simulink model "MPC_mobile_base_KIN"  (R2018b)
settings: Solver=ode4  StartTime=0.0  StopTime=inf  FixedStep=Tsample  RelTol=1e-3
values from neighbouring files (symbols this model uses):
  N = 6    [MPC_kin_N=6arc traj.mat]    (also in MPC_kin_N=7complex traj_ultimo.mat = 7; MPC_kin_Param_N=10 traj_retta.mat = 10; MPC_kin_Param_N=10 traj_ultimo.mat = 10; Traj_Prova.m = 5)
  p_0 = [0 0 0 0 0 0 0]    [MPC_kin_Param_N=10 traj_retta.mat]    (also in MPC_kin_Param_N=10 traj_ultimo.mat; Traj_Prova.m = zeros(1,7); traiettoria2.m = zeros(1,7); untitled5.m = zeros(1,7))
  T = 0.5    [MPC_kin_N=6arc traj.mat]    (also in MPC_kin_N=7complex traj_ultimo.mat = 0.2; MPC_kin_Param_N=10 traj_retta.mat = 0.4; MPC_kin_Param_N=10 traj_ultimo.mat = 0.4; Traj_Prova.m = 0.2)
  Tsample = 0.01    [MPC_kin_N=6arc traj.mat]    (also in MPC_kin_N=7complex traj_ultimo.mat; MPC_kin_Param_N=10 traj_retta.mat; MPC_kin_Param_N=10 traj_ultimo.mat = 0.08; Traj_Prova.m)
  xd = [0 0 0 0 0 0.000654498469498 0.0758636207458 4.96526307585e-05 0.00261799387799 0.227590374774 0.000446873251435 0.00589048622548 ... (153 elements, 3x51)]    [MPC_kin_N=6arc traj.mat]    (also in MPC_kin_N=7complex traj_ultimo.mat = [0 0 0 0.1 0 0 0.2 0 0 0.3 0 0 ... (303 elements, 3x101)]; MPC_kin_Param_N=10 traj_retta.mat = [0 2 0.785398163397 0.08 2.08 0.785398163397 0.16 2.16 0.785; MPC_kin_Param_N=10 traj_ultimo.mat = [0 2 0.785398163397 0.016 2.016 0.785398163397 0.032 2.032 0; Traj_Prova.m = [xdx; xdy; xdth])
undefined symbols (not defined in the file or in its folder): DiscIntNeverNeededParam
libraries: simulink x3, templibrary x1
settings Model: Creator=RaffaelePC  LastModifiedBy=Francesco Gennari
settings DebuggingCC: UnderSpecifiedDimensionMsg=warning

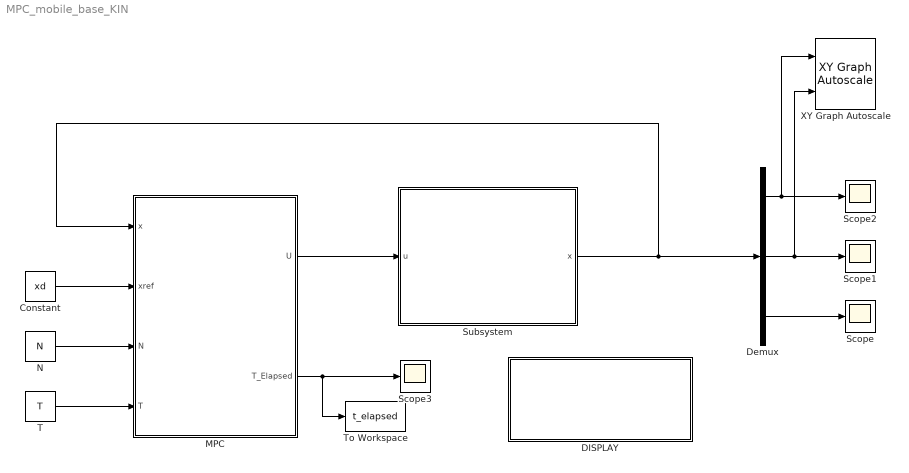
== system MPC_mobile_base_KIN ==
  Constant : Constant  Value=xd
  DISPLAY : Subsystem
  Demux : Demux  Outputs=3
  MPC : Subsystem
      mask Display: fprintf('MPC CONTROLLER')
  N : Constant  Value=N
  Scope{,1..3} (4 alike) : Scope
  Subsystem : Subsystem
      mask Display: disp('{\bf\fontsize{10}KINEMATIC SYSTEM}', 'texmode','on');
  T : Constant  Value=T
  To Workspace : ToWorkspace  VariableName=t_elapsed  SampleTime=T
      settings: Save2DSignal=2-D array (concatenate along first dimension)
  XY Graph Autoscale : templibrary/XY Graph  Autoscale  xmin=-1  xmax=1  ymin=-1  ymax=1  st=-1
  wires:
  N/1 -> MPC/3(N)
  T/1 -> MPC/4(T)
  Constant/1 -> MPC/2(xref)
  Subsystem/1(x) -> Demux/1, MPC/1(x)
  Demux/3 -> Scope/1
  Demux/1 -> XY Graph Autoscale/1, Scope2/1
  Demux/2 -> XY Graph Autoscale/2, Scope1/1
  MPC/2(T_Elapsed) -> To Workspace/1, Scope3/1
  MPC/1(U) -> Subsystem/1(u)

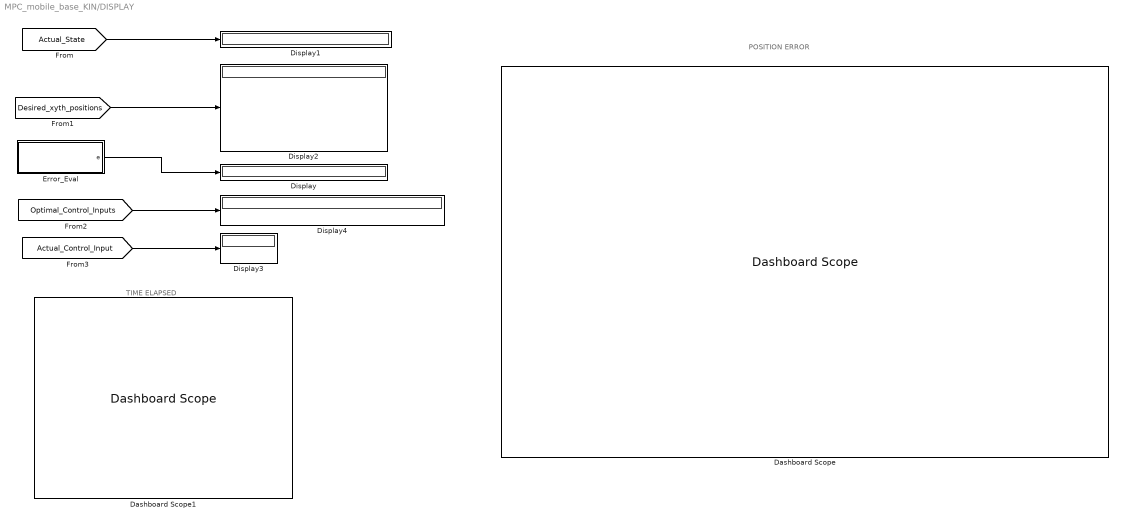
== system MPC_mobile_base_KIN/DISPLAY ==
  note: POSITION ERROR
  note: TIME ELAPSED
  Dashboard Scope : DashboardScope  WebBlockId=507  Ymin=-0.5  Ymax=0.5
  Dashboard Scope1 : DashboardScope  WebBlockId=516  Ymin=0  Ymax=1
  Display{,1..4} (5 alike) : Display
  "Error_Eval " : Subsystem
  wires:
  [Optimal_Control_Inputs] -> Display4/1
  [Desired_xyth_positions] -> Display2/1
  [Actual_Control_Input] -> Display3/1
  [Actual_State] -> Display1/1
  "Error_Eval "/1(e) -> Display/1

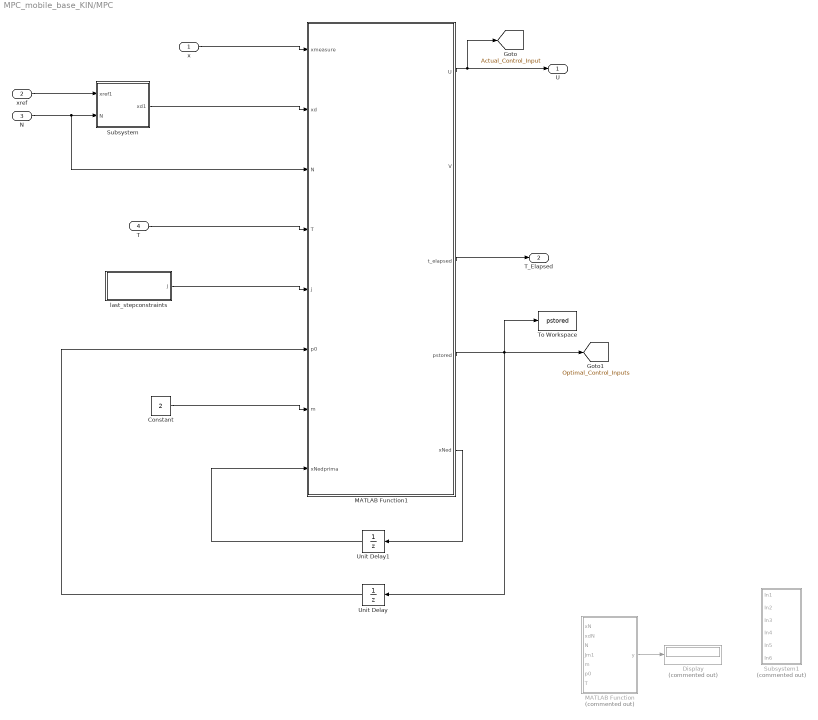
== system MPC_mobile_base_KIN/MPC ==
  x : Inport
  xref : Inport  Port=2
  N : Inport  Port=3
  T : Inport  Port=4
  Constant : Constant  Value=2
  Display : Display  Commented=on
  MATLAB Function : MATLAB Function  Commented=on  TreatAsAtomicUnit=on
  MATLAB Function1 : MATLAB Function  TreatAsAtomicUnit=on
  Subsystem : Subsystem
  Subsystem1 : Subsystem  Commented=on
  To Workspace : ToWorkspace  VariableName=pstored  SampleTime=-1
      settings: Save2DSignal=2-D array (concatenate along first dimension)
  Unit Delay : UnitDelay  InitialCondition=[0 0 0 0 0 0 N]  SampleTime=-1
  Unit Delay1 : UnitDelay  InitialCondition=zeros(2,3)  SampleTime=-1
  last_stepconstraints : Subsystem
  U : Outport
  T_Elapsed : Outport  Port=2
  tag scope: Actual_Control_Input=global, Optimal_Control_Inputs=global
  wires:
  Subsystem/1(xd1) -> MATLAB Function1/2(xd)
  MATLAB Function1/1(U) -> [Actual_Control_Input], U/1
  MATLAB Function1/4(pstored) -> [Optimal_Control_Inputs], To Workspace/1, Unit Delay/1
  Unit Delay/1 -> MATLAB Function1/6(p0)
  xref/1 -> Subsystem/1(xref1)
  x/1 -> MATLAB Function1/1(xmeasure)
  N/1 -> MATLAB Function1/3(N), Subsystem/2(N)
  T/1 -> MATLAB Function1/4(T)
  last_stepconstraints/1(j) -> MATLAB Function1/5(j)
  MATLAB Function1/3(t_elapsed) -> T_Elapsed/1
  MATLAB Function/1(y) -> Display/1
  Constant/1 -> MATLAB Function1/7(m)
  MATLAB Function1/5(xNed) -> Unit Delay1/1
  Unit Delay1/1 -> MATLAB Function1/8(xNedprima)

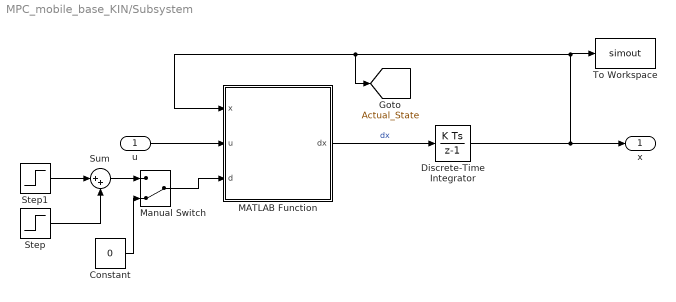
== system MPC_mobile_base_KIN/Subsystem ==
  u : Inport
  Constant : Constant  Value=0
  Discrete-Time Integrator : DiscreteIntegrator  InitialCondition=[0 0 0]  SampleTime=-1  ICPrevOutput=DiscIntNeverNeededParam  ICPrevScaledInput=DiscIntNeverNeededParam
  MATLAB Function : MATLAB Function  TreatAsAtomicUnit=on
  Manual Switch : ManualSwitch  CurrentSetting=0
  Step : Step  Time=100  SampleTime=Tsample
  Step1 : Step  Time=104  After=-1  SampleTime=Tsample
  Sum : Sum  Inputs=|++
  To Workspace : ToWorkspace  VariableName=simout  SaveFormat=Timeseries  SampleTime=-1
  x : Outport
  tag scope: Actual_State=global
  wires:
  u/1 -> MATLAB Function/2(u)
  MATLAB Function/1(dx) -> Discrete-Time Integrator/1  "dx"
  Discrete-Time Integrator/1 -> [Actual_State], MATLAB Function/1(x), To Workspace/1, x/1
  Step1/1 -> Sum/1
  Step/1 -> Sum/2
  Sum/1 -> Manual Switch/1
  Manual Switch/1 -> MATLAB Function/3(d)
  Constant/1 -> Manual Switch/2

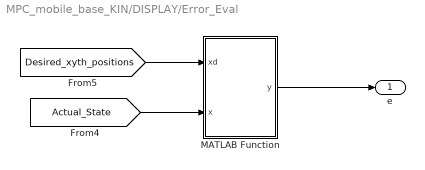
== system MPC_mobile_base_KIN/DISPLAY/Error_Eval  ==
  MATLAB Function : MATLAB Function  TreatAsAtomicUnit=on
  e : Outport
  wires:
  MATLAB Function/1(y) -> e/1
  [Desired_xyth_positions] -> MATLAB Function/1(xd)
  [Actual_State] -> MATLAB Function/2(x)

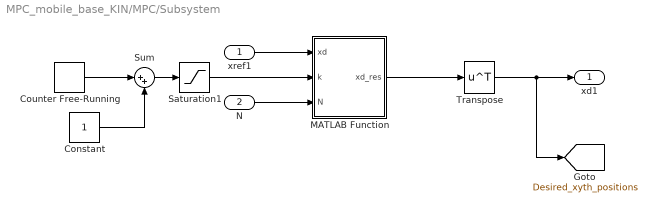
== system MPC_mobile_base_KIN/MPC/Subsystem ==
  xref1 : Inport
  N : Inport  Port=2
  Constant : Constant
  Counter Free-Running : simulink/Sources/Counter Free-Running  NumBits=12  tsamp=-1
  MATLAB Function : MATLAB Function  TreatAsAtomicUnit=on
  Saturation1 : Saturate  UpperLimit=size(xd,2)
  Sum : Sum  Inputs=|++
  Transpose : Math  Operator=transpose  SaturateOnIntegerOverflow=on
  xd1 : Outport
  tag scope: Desired_xyth_positions=global
  wires:
  Transpose/1 -> [Desired_xyth_positions], xd1/1
  MATLAB Function/1(xd_res) -> Transpose/1
  N/1 -> MATLAB Function/3(N)
  xref1/1 -> MATLAB Function/1(xd)
  Constant/1 -> Sum/2
  Counter Free-Running/1 -> Sum/1
  Sum/1 -> Saturation1/1
  Saturation1/1 -> MATLAB Function/2(k)

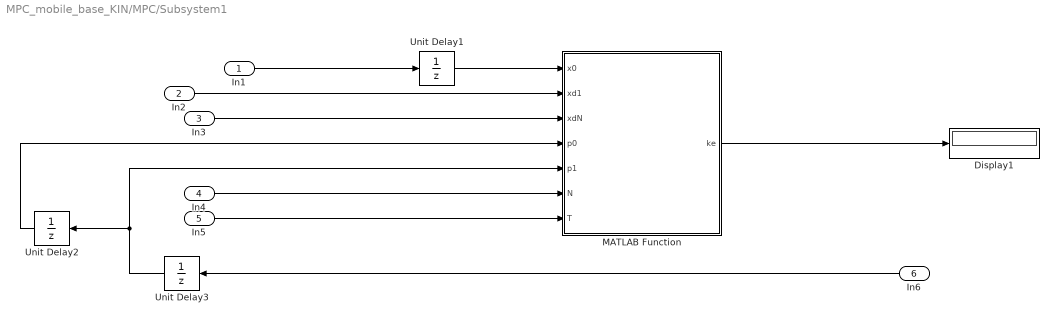
== system MPC_mobile_base_KIN/MPC/Subsystem1 ==
  In1 : Inport
  In2 : Inport  Port=2
  In3 : Inport  Port=3
  In4 : Inport  Port=4
  In5 : Inport  Port=5
  In6 : Inport  Port=6
  Display1 : Display
  MATLAB Function : MATLAB Function  TreatAsAtomicUnit=on
  Unit Delay1 : UnitDelay  InitialCondition=zeros(1,3)  SampleTime=-1
  Unit Delay2 : UnitDelay  InitialCondition=zeros(size(p_0))  SampleTime=-1
  Unit Delay3 : UnitDelay  InitialCondition=zeros(size(p_0))  SampleTime=-1
  wires:
  In4/1 -> MATLAB Function/6(N)
  Unit Delay1/1 -> MATLAB Function/1(x0)
  Unit Delay2/1 -> MATLAB Function/4(p0)
  In3/1 -> MATLAB Function/3(xdN)
  In5/1 -> MATLAB Function/7(T)
  MATLAB Function/1(ke) -> Display1/1
  In6/1 -> Unit Delay3/1
  In1/1 -> Unit Delay1/1
  In2/1 -> MATLAB Function/2(xd1)
  Unit Delay3/1 -> MATLAB Function/5(p1), Unit Delay2/1

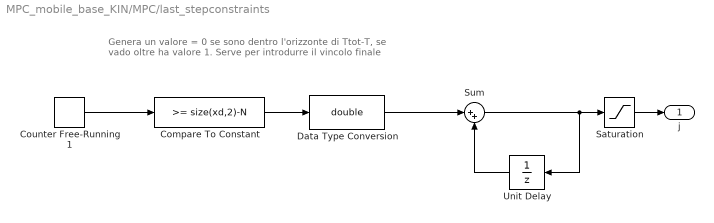
== system MPC_mobile_base_KIN/MPC/last_stepconstraints ==
  note: Genera un valore = 0 se sono dentro l'orizzonte di Ttot-T, se vado oltre ha valore 1. Serve per introdurre il vincolo finale
  Compare To Constant : simulink/Logic and Bit Operations/Compare To Constant  relop=>=  const=size(xd,2)-N  OutDataTypeStr=boolean
  Counter Free-Running1 : simulink/Sources/Counter Free-Running  NumBits=12  tsamp=-1
  Data Type Conversion : DataTypeConversion  OutDataTypeStr=double
  Saturation : Saturate  UpperLimit=N
  Sum : Sum  Inputs=|++
  Unit Delay : UnitDelay  SampleTime=-1
  j : Outport
  wires:
  Compare To Constant/1 -> Data Type Conversion/1
  Counter Free-Running1/1 -> Compare To Constant/1
  Sum/1 -> Unit Delay/1, Saturation/1
  Data Type Conversion/1 -> Sum/1
  Unit Delay/1 -> Sum/2
  Saturation/1 -> j/1

== matlab function MPC_mobile_base_KIN/MPC/Subsystem1/MATLAB Function ==
  data: x0 input size=[1 3]; xd1 input size=[3 1]; xdN input size=[3 1]; p0 input size=[size(p_0)]; p1 input size=[size(p_0)]; N input size=[1]; T input size=[1]; ke output size=[1]
function ke  = m_evaluationfunction(x0,xd1,xdN,p0,p1,N,T)
coder.extrinsic('m_evaluation')

m=0;
ke=0;

xd1=xd1.';
xdN=xdN.';


[ke] = m_evaluation(x0,xd1,xdN,p0,p1,N,T);

end

== matlab function MPC_mobile_base_KIN/MPC/Subsystem/MATLAB Function ==
  settings: updateMethod=DISCRETE  sampleTime=T
  data: xd input; xd_res output size=[3 N+1]; k input; N input
function xd_res   = fcn(xd,k,N)

if size(xd,2)-k>=N
h=xd(:,k:k+N);
xd_res=h;

      
else
h=[xd(:,k:end) xd(:,end)*ones(1,N-(size(xd,2)-k))];
xd_res = h;

end

== matlab function MPC_mobile_base_KIN/MPC/MATLAB Function1 ==
  settings: updateMethod=DISCRETE  sampleTime=T
  data: xmeasure input size=3; U output size=[2 1]; V output size=[1]; t_elapsed output double size=[1]; xd input; N input; T input; j input; p0 input size=[size(p_0)]; pstored output double size=[size(p_0)] [..20]; xNed output size=[2 3]; m input; xNedprima input size=[2 3]
function [U,V,t_elapsed,pstored,xNed] = MPC(xmeasure,xd,N,T,j,p0,m,xNedprima)
coder.extrinsic('tic')
coder.extrinsic('toc')
coder.extrinsic('MPCSOLVER_KIN');
coder.extrinsic('controlaction_out');

xNed=zeros(2,3);
V=0;

xN=zeros(1,3);

t_elapsed=0;

t_start=tic;

U=zeros(2,1);
xs=xd;

pstored=p0;

    %% dati solutore


% options = optimset('Display','off',...
%                 'TolFun', 1e-6,...
%                 'MaxIter', 10000,...
%                 'Algorithm', 'active-set',...
%                 'FinDiffType', 'forward',...
%                 'RelLineSrchBnd', [],...
%                 'RelLineSrchBndDuration', 1,...
%                 'TolConSQP', 1e-6);

%% MPC ALGORITHM 

x0=xmeasure';
t0=0;

if size(xd,1)<N
% tt=[];
%     for k=1:N
%         
%     tt(k)=T*(k-1);
%    
%     u_new(1,k) = tretratti(tt(k),N*T,p0,T);
%     u_new(2,k) = p0(4)*tt(k)^3+p0(5)*tt(k)^2+p0(6)*tt(k)+p0(7);
%     
%     end
%     U=u_new(:,1);
%     
%     pstored=p0;
    
else
    
   

    [p_new, V, xN] = MPCSOLVER_KIN(N, t0, x0, p0, T, xs, xd,j,m,xNedprima);

%   [u_new, V] = solveOptimalControlProblem ...
%         (@runningcosts, @terminalcosts, @constraints, @terminalconstraints, ...
%         @linearconstraints, @system, N, t0, x0, u0, T, xs, xd);
     
    pstored=p_new;
    
    [u_new] = controlaction_out(T,N,p_new,xN,xd(end,:));

    U(1,1)=u_new(1,1);
    U(2,1)=u_new(2,1);
    
    xNed(1,:)=xN;
    xNed(2,:)=xd(end,:);
    
    
t_elapsed=toc(t_start);




end 

end

== matlab function MPC_mobile_base_KIN/DISPLAY/Error_Eval /MATLAB Function ==
  settings: updateMethod=DISCRETE  sampleTime=T
  data: xd input; y output size=[3 1]; x input
function y = fcn(xd,x)

h = [xd(1,1)-x(1);xd(1,2)-x(2);xd(1,3)-x(3)];
y=h;

== matlab function MPC_mobile_base_KIN/MPC/MATLAB Function ==
  data: xN input; y output size=[1]; xdN input; N input; Jm1 input; m input; p0 input; T input
function y = fcn(xN,xdN,N,Jm1,m,p0,T)

coder.extrinsic('system_out')
 xNp=zeros(1,3);

u=zeros(2,1);

xs=xdN;

Q=eye(size(xs,2))*400;

 tt=T*(N-1);
    
u(1) = p0(1)*tt^2+p0(2)*tt+p0(3);  %tretratti(tt(k),N*T,p,T);
u(2) = p0(4)*tt^2+p0(5)*tt+p0(6);


    xNp(1,1)=xN(1)+T*u(1,1)*cos(xN(3));
    xNp(1,2)=xN(2)+T*u(1,1)*sin(xN(3));
    xNp(1,3)=xN(3)+T*u(2,1);

lf=([xNp(1)-xs(1) xNp(2)-xs(2) xNp(3)-xs(3)])*Q*([xNp(1)-xs(1) xNp(2)-xs(2) xNp(3)-xs(3)]).';

phi=1-((N-1)/N).^m;

y = phi*Jm1-lf;

== matlab function MPC_mobile_base_KIN/Subsystem/MATLAB Function ==
  settings: updateMethod=DISCRETE  sampleTime=T
  data: x input; dx output; u input size=[2 1]; d input
function dx = sys_dynamics(x,u,d)
dx=zeros(1,3);
dx(1,1)=u(1,1)*cos(x(3))+d;
dx(1,2)=u(1,1)*sin(x(3))+d;
dx(1,3)=u(2,1)-0.1*d;

end
